simulink model "state_space_model_v001"  (R2022b)
settings: Solver=VariableStepAuto  StartTime=0.0  StopTime=20  RelTol=1e-3
undefined symbols (not defined in the file): A_hat, A_num, b_hat, b_num, C, DiscIntNeverNeededParam, F, F_new, init_cond, Ts
settings Model: NumberOfSteps=10  Creator=ninj2  LastModifiedBy=ninj2
settings DebuggingCC: UnconnectedInputMsg=warning  UnconnectedOutputMsg=warning  UnconnectedLineMsg=warning
settings ModelReferenceCC: EnableRefExpFcnMdlSchedulingChecks=on
settings RTWCC: DLArmComputeVersion=19.05

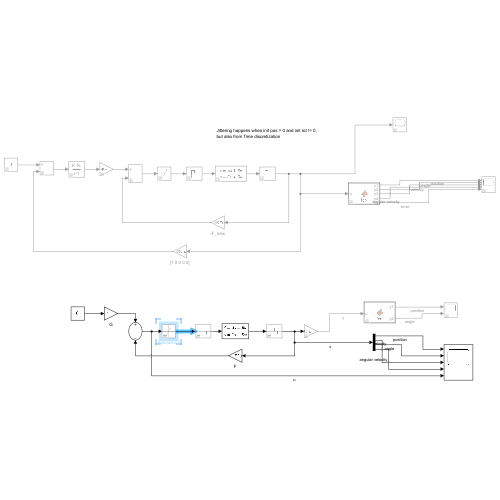
[thumbnail: Simulink's stored preview of the top-level diagram]
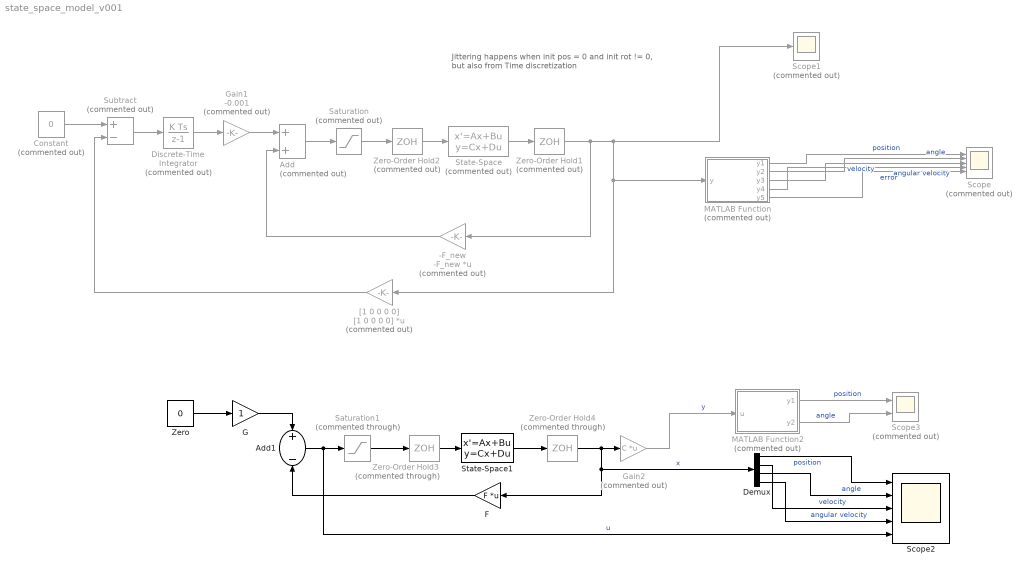
== system state_space_model_v001 ==
  note: Jittering happens when init pos = 0 and init rot != 0,
      | but also from Time discretization
  -F_new : Gain  Commented=on  Gain=-F_new  Multiplication=Matrix(K*u)
  Add : Sum  Commented=on
  Add1 : Sum  Inputs=+-
  Constant : Constant  Commented=on  Value=0
  Demux : Demux
  Discrete-Time Integrator : DiscreteIntegrator  Commented=on  SampleTime=Ts  ICPrevOutput=DiscIntNeverNeededParam  ICPrevScaledInput=DiscIntNeverNeededParam
  F : Gain  Gain=F  Multiplication=Matrix(K*u)
  G : Gain
  Gain1 : Gain  Commented=on  Gain=-0.001
  Gain2 : Gain  Commented=on  Gain=C  Multiplication=Matrix(K*u)
  MATLAB Function : MATLAB Function  Commented=on  TreatAsAtomicUnit=on
  MATLAB Function2 : MATLAB Function  Commented=on  TreatAsAtomicUnit=on
  Saturation : Saturate  Commented=on  UpperLimit=9  LowerLimit=-9  LinearizeAsGain=off
  Saturation1 : Saturate  Commented=through  UpperLimit=9  LowerLimit=-9
  Scope : Scope  Commented=on  NumInputPorts=5
  Scope1 : Scope  Commented=on
  Scope2 : Scope  NumInputPorts=5
  Scope3 : Scope  Commented=on  NumInputPorts=2
  State-Space : StateSpace  Commented=on  A=A_hat  B=b_hat  C=eye(5)  D=[0; 0; 0; 0;0]  InitialCondition=[init_cond 0]
  State-Space1 : StateSpace  A=A_num  B=b_num  C=eye(4)  D=[0; 0; 0; 0]  InitialCondition=init_cond
  Subtract : Sum  Commented=on  Inputs=+-
  Zero : Constant  Value=0  OutDataTypeStr=Inherit: Inherit via back propagation
  Zero-Order Hold1 : ZeroOrderHold  Commented=on  SampleTime=Ts
  Zero-Order Hold2 : ZeroOrderHold  Commented=on  SampleTime=Ts
  Zero-Order Hold3 : ZeroOrderHold  Commented=through  SampleTime=Ts
  Zero-Order Hold4 : ZeroOrderHold  Commented=through  SampleTime=Ts
  "[1 0 0 0 0]" : Gain  Commented=on  Gain=[1 0 0 0 0]  Multiplication=Matrix(K*u)
  wires:
  MATLAB Function/1(y1) -> Scope/1  "position"
  MATLAB Function/2(y2) -> Scope/2  "angle"
  MATLAB Function/3(y3) -> Scope/3  "velocity"
  MATLAB Function/4(y4) -> Scope/4  "angular velocity"
  State-Space/1 -> Zero-Order Hold1/1
  Zero-Order Hold1/1 -> -F_new/1, "[1 0 0 0 0]"/1, MATLAB Function/1(y), Scope1/1
  -F_new/1 -> Add/2
  Saturation/1 -> Zero-Order Hold2/1
  Zero-Order Hold2/1 -> State-Space/1
  Subtract/1 -> Discrete-Time Integrator/1
  "[1 0 0 0 0]"/1 -> Subtract/2
  Discrete-Time Integrator/1 -> Gain1/1
  Add/1 -> Saturation/1
  State-Space1/1 -> Zero-Order Hold4/1
  F/1 -> Add1/2
  Zero-Order Hold3/1 -> State-Space1/1
  Demux/1 -> Scope2/1  "position"
  Demux/3 -> Scope2/2  "angle"
  Demux/2 -> Scope2/3  "velocity"
  Demux/4 -> Scope2/4  "angular velocity"
  MATLAB Function/5(y5) -> Scope/5  "error"
  Gain1/1 -> Add/1
  Constant/1 -> Subtract/1
  Add1/1 -> Scope2/5, Saturation1/1  "u"
  Zero/1 -> G/1
  Gain2/1 -> MATLAB Function2/1(u)  "y"
  MATLAB Function2/1(y1) -> Scope3/1  "position"
  MATLAB Function2/2(y2) -> Scope3/2  "angle"
  Zero-Order Hold4/1 -> F/1, Demux/1, Gain2/1  "x"
  G/1 -> Add1/1
  Saturation1/1 -> Zero-Order Hold3/1

== matlab function state_space_model_v001/MATLAB Function ==
  data: y input; y1 output; y2 output; y3 output; y4 output; y5 output
function [y1, y2, y3, y4, y5]= fcn(y)

y1 = y(1);
y2 = y(2);
y3 = y(3);
y4 = y(4);
y5 = y(5);

== matlab function state_space_model_v001/MATLAB Function2 ==
  data: u input; y1 output; y2 output
function [y1, y2] = fcn(u)

y1 = u(1);
y2 = u(2);
